simulink subsystem "DAC"  (R2023a)
settings: Solver=VariableStepAuto  StartTime=0.0  StopTime=10.0  RelTol=1e-3
settings Model: Creator=motya  LastModifiedBy=motya

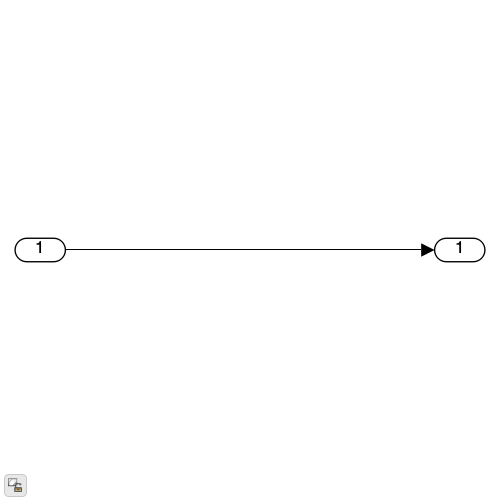
[thumbnail: Simulink's stored preview of the top-level diagram]
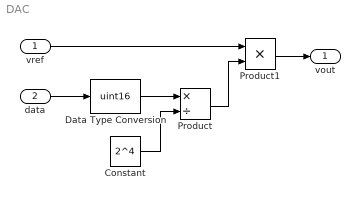
== system DAC ==
  vref : Inport
  data : Inport  Port=2
  Constant : Constant  Value=2^4
  Data Type Conversion : DataTypeConversion  OutDataTypeStr=uint16  RndMeth=Nearest  SaturateOnIntegerOverflow=off
  Product : Product  Inputs=*/
  Product1 : Product
  vout : Outport
  wires:
  Constant/1 -> Product/2
  Product/1 -> Product1/2
  vref/1 -> Product1/1
  Product1/1 -> vout/1
  Data Type Conversion/1 -> Product/1
  data/1 -> Data Type Conversion/1
